simulink model "PIDcontroller4"  (R2020b)
settings: Solver=ode4  StartTime=0.0  StopTime=10.0  FixedStep=0.01  RelTol=1e-3
model workspace (MAT data in the model file):
  D = Simulink.Parameter
  D.Value = 0.89767517
  D.DataType = 'auto'
  D.Dimensions = [1 1]
  I = Simulink.Parameter
  I.Value = 4810.143
  I.DataType = 'auto'
  I.Dimensions = [1 1]
  N = Simulink.Parameter
  N.Value = 119827
  N.DataType = 'auto'
  N.Dimensions = [1 1]
  P = Simulink.Parameter
  P.Value = 97.11869
  P.DataType = 'auto'
  P.Dimensions = [1 1]
settings Model: Creator=lalit  LastModifiedBy=lalit
settings DataIOCC: SaveOutput=off  SaveTime=off

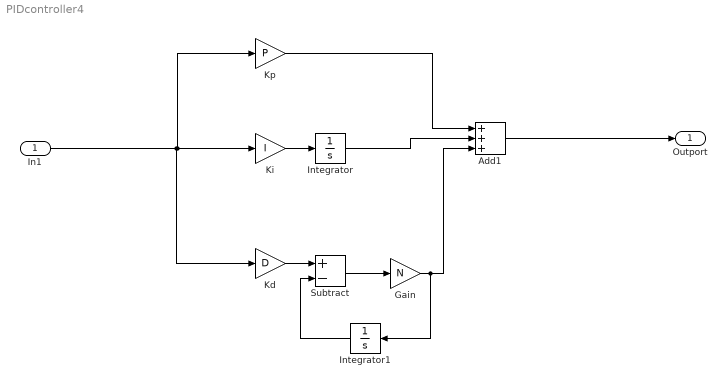
== system PIDcontroller4 ==
  In1 : Inport  OutDataTypeStr=double  PortDimensions=1  SampleTime=0
  Add1 : Sum  Inputs=+++
  Gain : Gain  Gain=N
  Integrator : Integrator
  Integrator1 : Integrator
  Kd : Gain  Gain=D
  Ki : Gain  Gain=I
  Kp : Gain  Gain=P
  Subtract : Sum  Inputs=+-
  Outport : Outport  OutDataTypeStr=double  PortDimensions=1  SampleTime=0
  wires:
  In1/1 -> Kd/1, Kp/1, Ki/1
  Kd/1 -> Subtract/1
  Integrator/1 -> Add1/2
  Add1/1 -> Outport/1
  Ki/1 -> Integrator/1
  Gain/1 -> Integrator1/1, Add1/3
  Kp/1 -> Add1/1
  Subtract/1 -> Gain/1
  Integrator1/1 -> Subtract/2
